simulink model "MBE_Simulation_04_Template_14_11_final"  (R2017b)
settings: Solver=FixedStepAuto  StartTime=0.0  StopTime=inf  FixedStep=0.05  RelTol=1e-3
libraries: simulink x67, canmsglib x4, instrumentlib x2, realtime_pacer_lib x1, hdlsllib x1
(part 2 of 4)

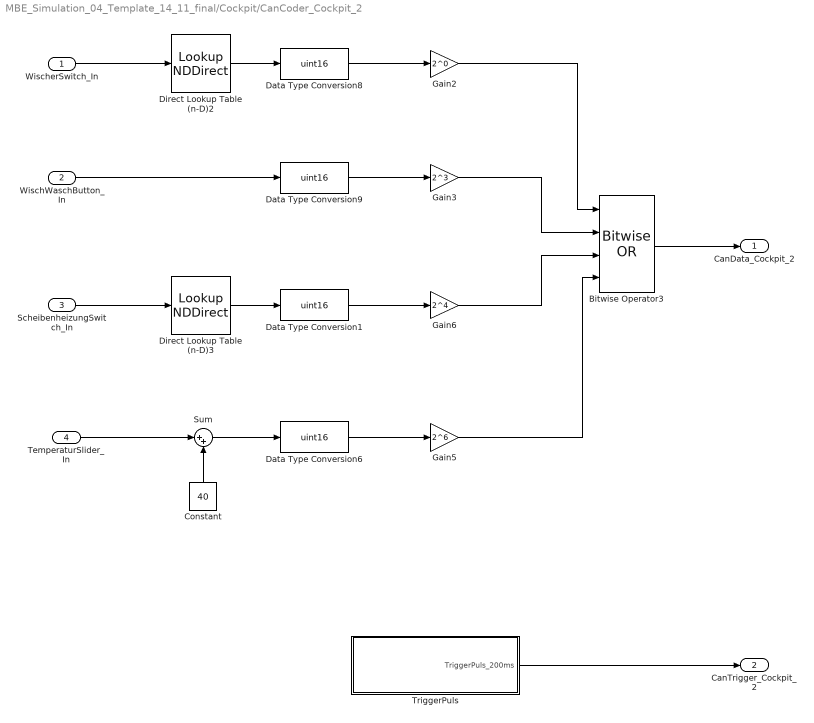
== system MBE_Simulation_04_Template_14_11_final/Cockpit/CanCoder_Cockpit_2 ==
  WischerSwitch_In : Inport
  WischWaschButton_In : Inport  Port=2
  ScheibenheizungSwitch_In : Inport  Port=3
  TemperaturSlider_In : Inport  Port=4
  Bitwise Operator3 : simulink/Logic and Bit Operations/Bitwise Operator  logicop=OR  UseBitMask=off  NumInputPorts=4  BitMask=bin2dec('11011001')  BitMaskRealWorld=Stored Integer
  Constant : Constant  Value=40  OutDataTypeStr=int16
  Data Type Conversion{1,6,8..9} (4 alike) : DataTypeConversion  OutDataTypeStr=uint16
  Direct Lookup Table (n-D)2 : LookupNDDirect  NumberOfTableDimensions=1  Table=[1; 0; 2; 3; 4; 5]
  Direct Lookup Table (n-D)3 : LookupNDDirect  NumberOfTableDimensions=1  Table=[1; 0; 2]
  Gain2 : Gain  Gain=2^0  OutDataTypeStr=uint16
  Gain3 : Gain  Gain=2^3  OutDataTypeStr=uint16
  Gain5 : Gain  Gain=2^6  OutDataTypeStr=uint16
  Gain6 : Gain  Gain=2^4  OutDataTypeStr=uint16
  Sum : Sum  Inputs=|++
  TriggerPuls : Subsystem
  CanData_Cockpit_2 : Outport
  CanTrigger_Cockpit_2 : Outport  Port=2
  wires:
  Data Type Conversion8/1 -> Gain2/1
  Sum/1 -> Data Type Conversion6/1
  Bitwise Operator3/1 -> CanData_Cockpit_2/1
  Data Type Conversion9/1 -> Gain3/1
  Constant/1 -> Sum/2
  Data Type Conversion6/1 -> Gain5/1
  Data Type Conversion1/1 -> Gain6/1
  Direct Lookup Table (n-D)2/1 -> Data Type Conversion8/1
  Direct Lookup Table (n-D)3/1 -> Data Type Conversion1/1
  Gain2/1 -> Bitwise Operator3/1
  Gain3/1 -> Bitwise Operator3/2
  Gain6/1 -> Bitwise Operator3/3
  Gain5/1 -> Bitwise Operator3/4
  ScheibenheizungSwitch_In/1 -> Direct Lookup Table (n-D)3/1
  TemperaturSlider_In/1 -> Sum/1
  WischWaschButton_In/1 -> Data Type Conversion9/1
  WischerSwitch_In/1 -> Direct Lookup Table (n-D)2/1
  TriggerPuls/1(TriggerPuls_200ms) -> CanTrigger_Cockpit_2/1

== system MBE_Simulation_04_Template_14_11_final/Cockpit/CanCoder_Cockpit_3 ==
  AlarmResetButton_In : Inport
  Detect Change4 : simulink/Logic and Bit Operations/Detect Change  vinit=0  OutDataTypeStr=boolean
  Gain : Gain  Gain=2^0  OutDataTypeStr=uint8
  CanData_Cockpit_3 : Outport
  CanTrigger_Cockpit_3 : Outport  Port=2
  wires:
  AlarmResetButton_In/1 -> Detect Change4/1, Gain/1
  Gain/1 -> CanData_Cockpit_3/1
  Detect Change4/1 -> CanTrigger_Cockpit_3/1

== system MBE_Simulation_04_Template_14_11_final/Cockpit/CanCoder_Cockpit_4 ==
  IgnitionSwitch_In : Inport
  Detect Change4 : simulink/Logic and Bit Operations/Detect Change  vinit=0  OutDataTypeStr=boolean
  Gain : Gain  Gain=2^0  OutDataTypeStr=uint8
  CanData_Cockpit_4 : Outport
  CanTrigger_Cockpit_4 : Outport  Port=2
  wires:
  Detect Change4/1 -> CanTrigger_Cockpit_4/1
  Gain/1 -> CanData_Cockpit_4/1
  IgnitionSwitch_In/1 -> Gain/1, Detect Change4/1

== system MBE_Simulation_04_Template_14_11_final/Cockpit/CanTransmit_Bremse_1 ==
  CanData_Bremse_1_In : Inport
  CanTrigger_Bremse_1_In : Inport  Port=2
  Bus Creator6 : BusCreator  Inputs=2
  CanTrigger_Bremse_1_Out : Outport
  wires:
  CanData_Bremse_1_In/1 -> Bus Creator6/1
  Bus Creator6/1 -> CanTrigger_Bremse_1_Out/1  "CanMsg_Bremse_1"
  CanTrigger_Bremse_1_In/1 -> Bus Creator6/2

== system MBE_Simulation_04_Template_14_11_final/Cockpit/CanTransmit_Bremse_2 ==
  CanData_Bremse_2_In : Inport
  CanTrigger_Bremse_2_In : Inport  Port=2
  Bus Creator3 : BusCreator  Inputs=2
  CanMsg_Bremse_2_Out : Outport
  wires:
  CanData_Bremse_2_In/1 -> Bus Creator3/1
  CanTrigger_Bremse_2_In/1 -> Bus Creator3/2
  Bus Creator3/1 -> CanMsg_Bremse_2_Out/1  "CanMsg_Bremse_2"

== system MBE_Simulation_04_Template_14_11_final/Cockpit/CanTransmit_Cockpit_1 ==
  CanData_Cockpit_1_In : Inport
  CanTrigger_Cockpit_1_In : Inport  Port=2
  Bus Creator : BusCreator  Inputs=2
  CanMsg_Cockpit_1_Out : Outport
  wires:
  CanData_Cockpit_1_In/1 -> Bus Creator/1
  CanTrigger_Cockpit_1_In/1 -> Bus Creator/2
  Bus Creator/1 -> CanMsg_Cockpit_1_Out/1  "CanMsg_Cockpit_1"

== system MBE_Simulation_04_Template_14_11_final/Cockpit/CanTransmit_Cockpit_2 ==
  CanData_Cockpit_2_In : Inport
  CanTrigger_Cockpit_2_In : Inport  Port=2
  Bus Creator1 : BusCreator  Inputs=2
  CanMsg_Cockpit_2_Out : Outport
  wires:
  CanData_Cockpit_2_In/1 -> Bus Creator1/1
  CanTrigger_Cockpit_2_In/1 -> Bus Creator1/2
  Bus Creator1/1 -> CanMsg_Cockpit_2_Out/1  "CanMsg_Cockpit_2"

== system MBE_Simulation_04_Template_14_11_final/Cockpit/CanTransmit_Cockpit_3 ==
  CanData_Cockpit_3_In : Inport
  CanTrigger_Cockpit_3_In : Inport  Port=2
  Bus Creator2 : BusCreator  Inputs=2
  CanMsg_Cockpit_3_Out : Outport
  wires:
  CanData_Cockpit_3_In/1 -> Bus Creator2/1
  CanTrigger_Cockpit_3_In/1 -> Bus Creator2/2
  Bus Creator2/1 -> CanMsg_Cockpit_3_Out/1  "CanMsg_Cockpit_3"

== system MBE_Simulation_04_Template_14_11_final/Cockpit/CanTransmit_Cockpit_4 ==
  CanData_Cockpit_4_In : Inport
  CanTrigger_Cockpit_4_In : Inport  Port=2
  Bus Creator5 : BusCreator  Inputs=2
  CanMsg_Cockpit_4_Out : Outport
  wires:
  CanData_Cockpit_4_In/1 -> Bus Creator5/1
  CanTrigger_Cockpit_4_In/1 -> Bus Creator5/2
  Bus Creator5/1 -> CanMsg_Cockpit_4_Out/1  "CanMsg_Cockpit_4"

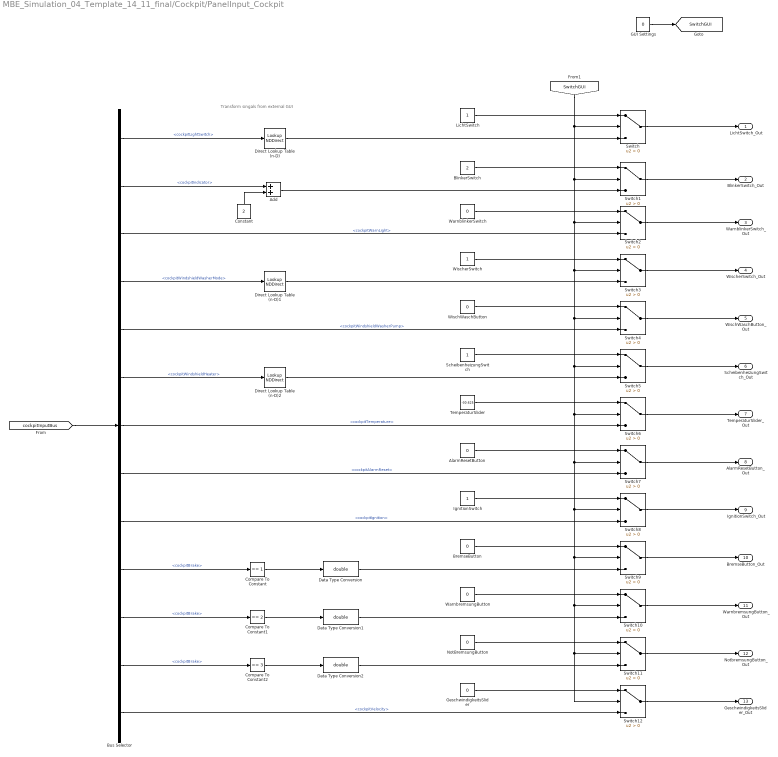
== system MBE_Simulation_04_Template_14_11_final/Cockpit/PanelInput_Cockpit ==
  note: Transform singals from external GUI
  Add : Sum
  AlarmResetButton : Constant  Value=0  OutDataTypeStr=uint8
  BlinkerSwitch : Constant  Value=2  OutDataTypeStr=uint8
  BremseButton : Constant  Value=0  OutDataTypeStr=uint8
  Bus Selector : BusSelector  OutputSignals=cockpitLightSwitch,cockpitIndicator,cockpitWarnLight,cockpitWindshieldWasherMode,cockpitWindshieldWasherPump,cockpitWindshieldHeater,cockpitTemperature,cockpitAlarmReset,cockpitIgnition,cockpitBrake,cockpitBrake,cockpitBrake,cockpitVelocity
  Compare To Constant : simulink/Logic and Bit Operations/Compare To Constant  relop===  const=1  OutDataTypeStr=boolean
  Compare To Constant1 : simulink/Logic and Bit Operations/Compare To Constant  relop===  const=2  OutDataTypeStr=boolean
  Compare To Constant2 : simulink/Logic and Bit Operations/Compare To Constant  relop===  const=3  OutDataTypeStr=boolean
  Constant : Constant  Value=2
  Data Type Conversion : DataTypeConversion  OutDataTypeStr=double
  Data Type Conversion1 : DataTypeConversion  OutDataTypeStr=double
  Data Type Conversion2 : DataTypeConversion  OutDataTypeStr=double
  Direct Lookup Table (n-D) : LookupNDDirect  NumberOfTableDimensions=1  Table=[1 0 2 3 4]
  Direct Lookup Table (n-D)1 : LookupNDDirect  NumberOfTableDimensions=1  Table=[1 0 2 3 4 5]
  Direct Lookup Table (n-D)2 : LookupNDDirect  NumberOfTableDimensions=1  Table=[1 0 2]
  GUI Settings : Constant  Value=0
  GeschwindigkeitsSlider : Constant  Value=0  OutDataTypeStr=uint8
  IgnitionSwitch : Constant  OutDataTypeStr=uint8
  LichtSwitch : Constant  OutDataTypeStr=uint8
  NotBremsungButton : Constant  Value=0  OutDataTypeStr=uint8
  ScheibenheizungSwitch : Constant  OutDataTypeStr=uint8
  Switch{,1..12} (13 alike) : Switch  Criteria=u2 > Threshold
  TemperaturSlider : Constant  Value=-30.625  OutDataTypeStr=int16
  WarnblinkerSwitch : Constant  Value=0  OutDataTypeStr=uint8
  WarnbremsungButton : Constant  Value=0  OutDataTypeStr=uint8
  WischWaschButton : Constant  Value=0  OutDataTypeStr=uint8
  WischerSwitch : Constant  OutDataTypeStr=uint8
  LichtSwitch_Out : Outport
  BlinkerSwitch_Out : Outport  Port=2
  WarnblinkerSwitch_Out : Outport  Port=3
  WischerSwitch_Out : Outport  Port=4
  WischWaschButton_Out : Outport  Port=5
  ScheibenheizungSwitch_Out : Outport  Port=6
  TemperaturSlider_Out : Outport  Port=7
  AlarmResetButton_Out : Outport  Port=8
  IgnitionSwitch_Out : Outport  Port=9
  BremseButton_Out : Outport  Port=10
  WarnbremsungButton_Out : Outport  Port=11
  NotbremsungButton_Out : Outport  Port=12
  GeschwindigkeitsSlider_Out : Outport  Port=13
  tag scope: SwitchGUI=global
  wires:
  [cockpitInputBus] -> Bus Selector/1
  Bus Selector/2 -> Add/1  "<cockpitIndicator>"
  Constant/1 -> Add/2
  Bus Selector/1 -> Direct Lookup Table (n-D)/1  "<cockpitLightSwitch>"
  Bus Selector/4 -> Direct Lookup Table (n-D)1/1  "<cockpitWindshieldWasherMode>"
  Bus Selector/10 -> Compare To Constant/1  "<cockpitBrake>"
  Bus Selector/6 -> Direct Lookup Table (n-D)2/1  "<cockpitWindshieldHeater>"
  Compare To Constant/1 -> Data Type Conversion/1
  Compare To Constant1/1 -> Data Type Conversion1/1
  Compare To Constant2/1 -> Data Type Conversion2/1
  Bus Selector/11 -> Compare To Constant1/1  "<cockpitBrake>"
  Bus Selector/12 -> Compare To Constant2/1  "<cockpitBrake>"
  Direct Lookup Table (n-D)/1 -> Switch/3
  Add/1 -> Switch1/3
  Bus Selector/3 -> Switch2/3  "<cockpitWarnLight>"
  Direct Lookup Table (n-D)1/1 -> Switch3/3
  Bus Selector/5 -> Switch4/3  "<cockpitWindshieldWasherPump>"
  Direct Lookup Table (n-D)2/1 -> Switch5/3
  Bus Selector/7 -> Switch6/3  "<cockpitTemperature>"
  Bus Selector/8 -> Switch7/3  "<cockpitAlarmReset>"
  Bus Selector/9 -> Switch8/3  "<cockpitIgnition>"
  Data Type Conversion/1 -> Switch9/3
  Data Type Conversion1/1 -> Switch10/3
  Data Type Conversion2/1 -> Switch11/3
  Bus Selector/13 -> Switch12/3  "<cockpitVelocity>"
  LichtSwitch/1 -> Switch/1
  BlinkerSwitch/1 -> Switch1/1
  WarnblinkerSwitch/1 -> Switch2/1
  WischerSwitch/1 -> Switch3/1
  WischWaschButton/1 -> Switch4/1
  ScheibenheizungSwitch/1 -> Switch5/1
  TemperaturSlider/1 -> Switch6/1
  AlarmResetButton/1 -> Switch7/1
  IgnitionSwitch/1 -> Switch8/1
  BremseButton/1 -> Switch9/1
  WarnbremsungButton/1 -> Switch10/1
  NotBremsungButton/1 -> Switch11/1
  GeschwindigkeitsSlider/1 -> Switch12/1
  Switch/1 -> LichtSwitch_Out/1
  Switch1/1 -> BlinkerSwitch_Out/1
  Switch2/1 -> WarnblinkerSwitch_Out/1
  Switch3/1 -> WischerSwitch_Out/1
  Switch4/1 -> WischWaschButton_Out/1
  Switch5/1 -> ScheibenheizungSwitch_Out/1
  Switch6/1 -> TemperaturSlider_Out/1
  Switch7/1 -> AlarmResetButton_Out/1
  Switch8/1 -> IgnitionSwitch_Out/1
  Switch9/1 -> BremseButton_Out/1
  Switch10/1 -> WarnbremsungButton_Out/1
  Switch11/1 -> NotbremsungButton_Out/1
  Switch12/1 -> GeschwindigkeitsSlider_Out/1
  [SwitchGUI] -> Switch/2, Switch1/2, Switch2/2, Switch3/2, Switch4/2, Switch5/2, Switch6/2, Switch7/2, Switch8/2, Switch9/2, Switch10/2, Switch11/2, Switch12/2
  GUI Settings/1 -> [SwitchGUI]

== system MBE_Simulation_04_Template_14_11_final/Dashboard/Gauge ==

== system MBE_Simulation_04_Template_14_11_final/Dashboard/Lamp ==

== system MBE_Simulation_04_Template_14_11_final/Dashboard/Lamp1 ==

== system MBE_Simulation_04_Template_14_11_final/Dashboard/Lamp10 ==

== system MBE_Simulation_04_Template_14_11_final/Dashboard/Lamp11 ==

== system MBE_Simulation_04_Template_14_11_final/Dashboard/Lamp12 ==

== system MBE_Simulation_04_Template_14_11_final/Dashboard/Lamp13 ==

== system MBE_Simulation_04_Template_14_11_final/Dashboard/Lamp14 ==

== system MBE_Simulation_04_Template_14_11_final/Dashboard/Lamp15 ==

== system MBE_Simulation_04_Template_14_11_final/Dashboard/Lamp16 ==

== system MBE_Simulation_04_Template_14_11_final/Dashboard/Lamp17 ==

== system MBE_Simulation_04_Template_14_11_final/Dashboard/Lamp18 ==

== system MBE_Simulation_04_Template_14_11_final/Dashboard/Lamp2 ==

== system MBE_Simulation_04_Template_14_11_final/Dashboard/Lamp20 ==

== system MBE_Simulation_04_Template_14_11_final/Dashboard/Lamp3 ==

== system MBE_Simulation_04_Template_14_11_final/Dashboard/Lamp4 ==

== system MBE_Simulation_04_Template_14_11_final/Dashboard/Lamp5 ==

== system MBE_Simulation_04_Template_14_11_final/Dashboard/Lamp6 ==

== system MBE_Simulation_04_Template_14_11_final/Dashboard/Lamp7 ==

== system MBE_Simulation_04_Template_14_11_final/Dashboard/Lamp8 ==

== system MBE_Simulation_04_Template_14_11_final/Dashboard/Lamp9 ==

== system MBE_Simulation_04_Template_14_11_final/Dashboard/Push Button ==

== system MBE_Simulation_04_Template_14_11_final/Dashboard/Push Button1 ==

== system MBE_Simulation_04_Template_14_11_final/Dashboard/Push Button2 ==

== system MBE_Simulation_04_Template_14_11_final/Dashboard/Push Button4 ==

== system MBE_Simulation_04_Template_14_11_final/Dashboard/Push Button5 ==

== system MBE_Simulation_04_Template_14_11_final/Dashboard/Quarter Gauge ==

== system MBE_Simulation_04_Template_14_11_final/Dashboard/Rocker Switch ==

== system MBE_Simulation_04_Template_14_11_final/Dashboard/Rocker Switch6 ==

== system MBE_Simulation_04_Template_14_11_final/Dashboard/Rotary Switch ==

== system MBE_Simulation_04_Template_14_11_final/Dashboard/Rotary Switch1 ==

== system MBE_Simulation_04_Template_14_11_final/Dashboard/Rotary Switch2 ==

== system MBE_Simulation_04_Template_14_11_final/Dashboard/Rotary Switch3 ==

== system MBE_Simulation_04_Template_14_11_final/Dashboard/Slider ==

== system MBE_Simulation_04_Template_14_11_final/Dashboard/Slider1 ==

== system MBE_Simulation_04_Template_14_11_final/Dashboard/Slider2 ==

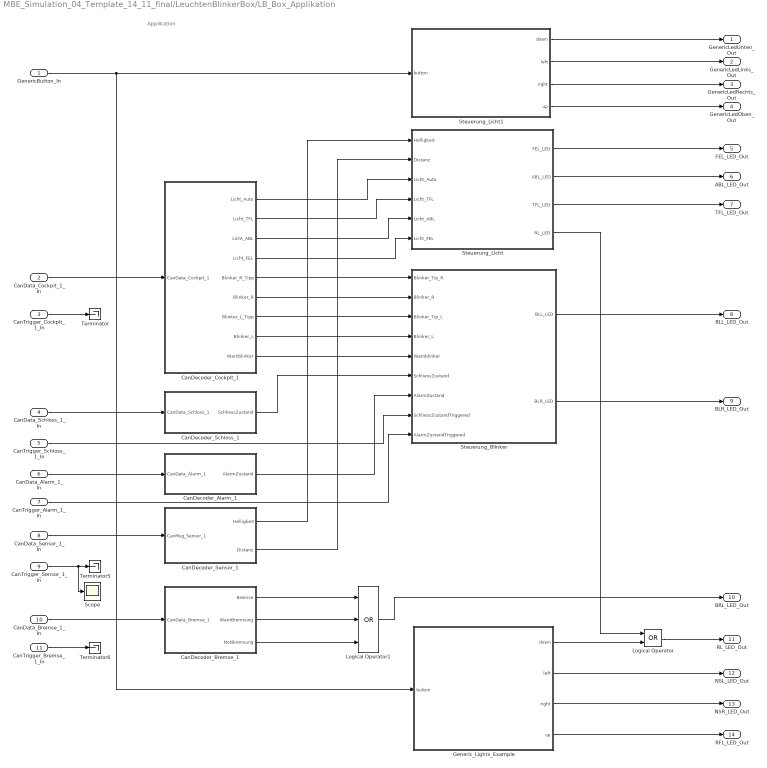
== system MBE_Simulation_04_Template_14_11_final/LeuchtenBlinkerBox/LB_Box_Applikation ==
  note: Applikation
  GenericButton_In : Inport
  CanData_Cockpit_1_In : Inport  Port=2
  CanTrigger_Cockpit_1_In : Inport  Port=3
  CanData_Schloss_1_In : Inport  Port=4
  CanTrigger_Schloss_1_In : Inport  Port=5
  CanData_Alarm_1_In : Inport  Port=6
  CanTrigger_Alarm_1_In : Inport  Port=7
  CanData_Sensor_1_In : Inport  Port=8
  CanTrigger_Sensor_1_In : Inport  Port=9
  CanData_Bremse_1_In : Inport  Port=10
  CanTrigger_Bremse_1_In : Inport  Port=11
  CanDecoder_Alarm_1 : Subsystem
  CanDecoder_Bremse_1 : Subsystem
  CanDecoder_Cockpit_1 : Subsystem
  CanDecoder_Schloss_1 : Subsystem
  CanDecoder_Sensor_1 : Subsystem
  Generic_Lights_Example : Stateflow chart  TreatAsAtomicUnit=on
  Logical Operator : Logic  Operator=OR  AllPortsSameDT=off  OutDataTypeStr=boolean
  Logical Operator1 : Logic  Operator=OR  Inputs=3  AllPortsSameDT=off  OutDataTypeStr=boolean
  Scope : Scope
  Steuerung_Blinker : Stateflow chart  TreatAsAtomicUnit=on
  Steuerung_Licht : Stateflow chart  TreatAsAtomicUnit=on
  Steuerung_Licht1 : Stateflow chart  TreatAsAtomicUnit=on
  Terminator : Terminator
  Terminator5 : Terminator
  Terminator6 : Terminator
  GenericLedUnten_Out : Outport
  GenericLedLinks_Out : Outport  Port=2
  GenericLedRechts_Out : Outport  Port=3
  GenericLedOben_Out : Outport  Port=4
  FEL_LED_Out : Outport  Port=5
  ABL_LED_Out : Outport  Port=6
  TFL_LED_Out : Outport  Port=7
  BLL_LED_Out : Outport  Port=8
  BLR_LED_Out : Outport  Port=9
  BRL_LED_Out : Outport  Port=10
  RL_LED_Out : Outport  Port=11
  NSL_LED_Out : Outport  Port=12
  NSR_LED_Out : Outport  Port=13
  RFL_LED_Out : Outport  Port=14
  wires:
  Steuerung_Blinker/2(BLR_LED) -> BLR_LED_Out/1
  Steuerung_Licht/2(ABL_LED) -> ABL_LED_Out/1
  Steuerung_Blinker/1(BLL_LED) -> BLL_LED_Out/1
  CanDecoder_Bremse_1/2(WarnBremsung) -> Logical Operator1/2
  CanDecoder_Cockpit_1/9(Warnblinker) -> Steuerung_Blinker/5(Warnblinker)
  CanDecoder_Cockpit_1/3(Licht_ABL) -> Steuerung_Licht/5(Licht_ABL)
  CanDecoder_Sensor_1/1(Helligkeit) -> Steuerung_Licht/1(Helligkeit)
  CanDecoder_Cockpit_1/4(Licht_FEL) -> Steuerung_Licht/6(Licht_FEL)
  CanDecoder_Cockpit_1/5(Blinker_R_Tipp) -> Steuerung_Blinker/1(Blinker_Tip_R)
  CanDecoder_Cockpit_1/8(Blinker_L) -> Steuerung_Blinker/4(Blinker_L)
  CanDecoder_Schloss_1/1(SchliessZustand) -> Steuerung_Blinker/6(SchliessZustand)
  CanDecoder_Alarm_1/1(AlarmZustand) -> Steuerung_Blinker/7(AlarmZustand)
  CanDecoder_Cockpit_1/1(Licht_Auto) -> Steuerung_Licht/3(Licht_Auto)
  CanDecoder_Cockpit_1/6(Blinker_R) -> Steuerung_Blinker/2(Blinker_R)
  CanDecoder_Cockpit_1/2(Licht_TFL) -> Steuerung_Licht/4(Licht_TFL)
  CanDecoder_Sensor_1/2(Distanz) -> Steuerung_Licht/2(Distanz)
  CanDecoder_Cockpit_1/7(Blinker_L_Tipp) -> Steuerung_Blinker/3(Blinker_Tip_L)
  CanData_Sensor_1_In/1 -> CanDecoder_Sensor_1/1(CanMsg_Sensor_1)
  CanData_Cockpit_1_In/1 -> CanDecoder_Cockpit_1/1(CanData_Cockpit_1)
  CanData_Schloss_1_In/1 -> CanDecoder_Schloss_1/1(CanData_Schloss_1)
  CanData_Alarm_1_In/1 -> CanDecoder_Alarm_1/1(CanData_Alarm_1)
  CanData_Bremse_1_In/1 -> CanDecoder_Bremse_1/1(CanData_Bremse_1)
  CanTrigger_Cockpit_1_In/1 -> Terminator/1
  CanTrigger_Schloss_1_In/1 -> Steuerung_Blinker/8(SchliessZustandTriggered)
  CanTrigger_Alarm_1_In/1 -> Steuerung_Blinker/9(AlarmZustandTriggered)
  CanTrigger_Sensor_1_In/1 -> Scope/1, Terminator5/1
  CanTrigger_Bremse_1_In/1 -> Terminator6/1
  Steuerung_Licht/1(FEL_LED) -> FEL_LED_Out/1
  Steuerung_Licht/3(TFL_LED) -> TFL_LED_Out/1
  Steuerung_Licht1/1(down) -> GenericLedUnten_Out/1
  Steuerung_Licht1/2(left) -> GenericLedLinks_Out/1
  Steuerung_Licht1/3(right) -> GenericLedRechts_Out/1
  Steuerung_Licht1/4(up) -> GenericLedOben_Out/1
  GenericButton_In/1 -> Generic_Lights_Example/1(button), Steuerung_Licht1/1(button)
  Generic_Lights_Example/1(down) -> Logical Operator/2
  Generic_Lights_Example/2(left) -> NSL_LED_Out/1
  Generic_Lights_Example/3(right) -> NSR_LED_Out/1
  Generic_Lights_Example/4(up) -> RFL_LED_Out/1
  CanDecoder_Bremse_1/3(NotBremsung) -> Logical Operator1/3
  Steuerung_Licht/4(RL_LED) -> Logical Operator/1
  Logical Operator/1 -> RL_LED_Out/1
  CanDecoder_Bremse_1/1(Bremse) -> Logical Operator1/1
  Logical Operator1/1 -> BRL_LED_Out/1

== system MBE_Simulation_04_Template_14_11_final/LeuchtenBlinkerBox/LB_Box_Simulation_Input ==
  CanBus_LB_In : Inport
  CanBus_Input : Subsystem
  CanReceive_Alarm_1 : Subsystem
  CanReceive_Bremse_1 : Subsystem
  CanReceive_Cockpit_1 : Subsystem
  CanReceive_Schloss_1 : Subsystem
  CanReceive_Sensor_1 : Subsystem
  GuiInput_LichtBox : Subsystem
  GenericButton_Out : Outport
  CanData_Cockpit_1_Out : Outport  Port=2
  CanTrigger_Cockpit_1_Out : Outport  Port=3
  CanData_Schloss_1_Out : Outport  Port=4
  CanTrigger_Schloss_1_Out : Outport  Port=5
  CanData_Alarm_1_Out : Outport  Port=6
  CanTrigger_Alarm_1_Out : Outport  Port=7
  CanData_Sensor_1_Out : Outport  Port=8
  CanTrigger_Sensor_1_Out : Outport  Port=9
  CanData_Bremse_1_Out : Outport  Port=10
  CanTrigger_Bremse_1_Out : Outport  Port=11
  wires:
  CanBus_LB_In/1 -> CanBus_Input/1(CanBus_LB_In)
  CanBus_Input/1(CanMsg_Cockpit_1_Out) -> CanReceive_Cockpit_1/1(CanData_Cockpit_1_In)
  CanBus_Input/2(CanMsg_Schloss_1_Out) -> CanReceive_Schloss_1/1(CanMsg_Schloss_1_In)
  CanBus_Input/3(CanMsg_Alarm_1_Out) -> CanReceive_Alarm_1/1(CanMsg_Alarm_1_In)
  CanBus_Input/4(CanMsg_Sensor_1_Out) -> CanReceive_Sensor_1/1(CanMsg_Sensor_1_In)
  CanBus_Input/5(CanMsg_Bremse_1_Out) -> CanReceive_Bremse_1/1(CanMsg_Bremse_1_In)
  CanReceive_Sensor_1/1(CanData_Sensor_1_Out) -> CanData_Sensor_1_Out/1
  CanReceive_Cockpit_1/2(CanTrigger_Cockpit_1_Out) -> CanTrigger_Cockpit_1_Out/1
  CanReceive_Alarm_1/1(CanData_Alarm_1_Out) -> CanData_Alarm_1_Out/1
  CanReceive_Schloss_1/2(CanTrigger_Schloss_1_Out) -> CanTrigger_Schloss_1_Out/1
  CanReceive_Bremse_1/1(CanData_Bremse_1_Out) -> CanData_Bremse_1_Out/1
  CanReceive_Bremse_1/2(CanTrigger_Bremse_1_Out) -> CanTrigger_Bremse_1_Out/1
  CanReceive_Schloss_1/1(CanData_Schloss_1_Out) -> CanData_Schloss_1_Out/1
  CanReceive_Cockpit_1/1(CanData_Cockpit_1_Out) -> CanData_Cockpit_1_Out/1
  CanReceive_Sensor_1/2(CanTrigger_Sensor_1_Out) -> CanTrigger_Sensor_1_Out/1
  CanReceive_Alarm_1/2(CanTrigger_Alarm_1_Out) -> CanTrigger_Alarm_1_Out/1
  GuiInput_LichtBox/1(GenericButton_Out) -> GenericButton_Out/1

== system MBE_Simulation_04_Template_14_11_final/LeuchtenBlinkerBox/LB_Box_Simulation_Output ==
  GenericLedUnten_LED_In : Inport
  GenericLedLinks_LED_In : Inport  Port=2
  GenericLedRechts_LED_In : Inport  Port=3
  GenericLedOben_LED_In : Inport  Port=4
  FEL_LED : Inport  Port=5
  ABL_LED : Inport  Port=6
  TFL_LED : Inport  Port=7
  BLL_LED : Inport  Port=8
  BLR_LED : Inport  Port=9
  BRL_LED : Inport  Port=10
  RL_LED : Inport  Port=11
  NSL_LED : Inport  Port=12
  NSR_LED : Inport  Port=13
  RFL_LED : Inport  Port=14
  Bus Creator : BusCreator  Inputs=14
  LeuchtenBlinkerLEDs : Subsystem
  tag scope: lightOutputBus=global
  wires:
  FEL_LED/1 -> Bus Creator/5, LeuchtenBlinkerLEDs/1(FEL_LED)
  ABL_LED/1 -> Bus Creator/6, LeuchtenBlinkerLEDs/2(ABL_LED)
  TFL_LED/1 -> Bus Creator/7, LeuchtenBlinkerLEDs/3(TFL_LED)
  BLL_LED/1 -> Bus Creator/8, LeuchtenBlinkerLEDs/4(BLL_LED)
  BLR_LED/1 -> Bus Creator/9, LeuchtenBlinkerLEDs/5(BLR_LED)
  BRL_LED/1 -> Bus Creator/10, LeuchtenBlinkerLEDs/6(BRL_LED)  "BRL_LED"
  Bus Creator/1 -> [lightOutputBus]
  GenericLedOben_LED_In/1 -> Bus Creator/4  "GenericLedOben"
  GenericLedRechts_LED_In/1 -> Bus Creator/3  "GenericLedRechts"
  GenericLedLinks_LED_In/1 -> Bus Creator/2  "GenericLedLinks"
  GenericLedUnten_LED_In/1 -> Bus Creator/1  "GenericLedUnten"
  RL_LED/1 -> Bus Creator/11  "RL_LED"
  NSL_LED/1 -> Bus Creator/12  "NSL_LED"
  NSR_LED/1 -> Bus Creator/13  "NSR_LED"
  RFL_LED/1 -> Bus Creator/14  "RFL_LED"

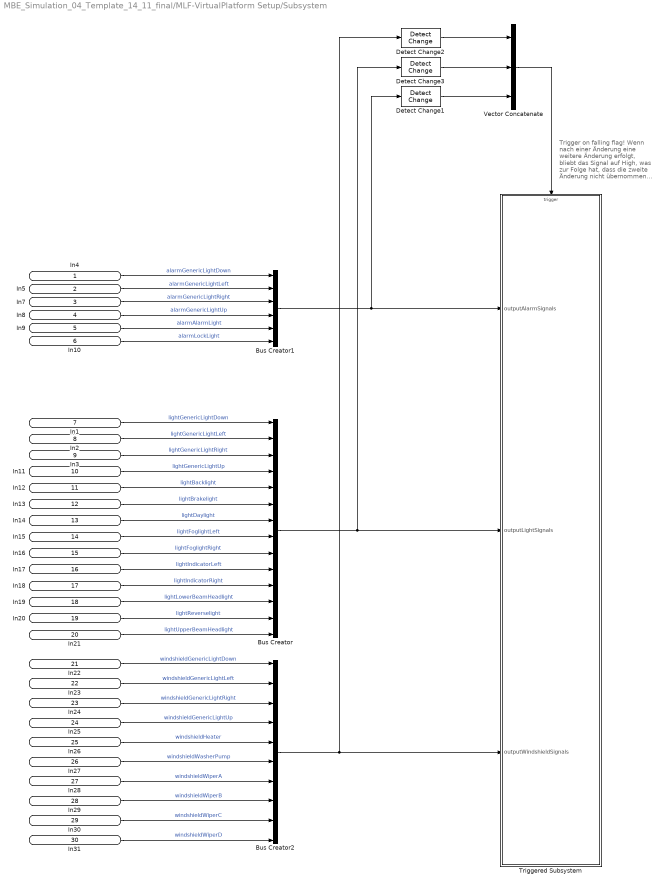
== system MBE_Simulation_04_Template_14_11_final/MLF-VirtualPlatform Setup/Subsystem ==
  note: Trigger on falling flag!
      | Wenn nach einer Änderung eine weitere Änderung erfolgt,
      | bliebt das Signal auf High, was zur Folge hat, dass die zweite
      | Änderung nicht übernommen wird. Durch das Triggern auf eine
      | fallende Flanke erfolgt das übertragen erst dann, wenn sich für
      | mindestens ein Zeitschritt ein konstanter Zustand eingestellt hat.
  In4 : Inport
  In5 : Inport  Port=2
  In7 : Inport  Port=3
  In8 : Inport  Port=4
  In9 : Inport  Port=5
  In10 : Inport  Port=6
  In1 : Inport  Port=7
  In2 : Inport  Port=8
  In3 : Inport  Port=9
  In11 : Inport  Port=10
  In12 : Inport  Port=11
  In13 : Inport  Port=12
  In14 : Inport  Port=13
  In15 : Inport  Port=14
  In16 : Inport  Port=15
  In17 : Inport  Port=16
  In18 : Inport  Port=17
  In19 : Inport  Port=18
  In20 : Inport  Port=19
  In21 : Inport  Port=20
  In22 : Inport  Port=21
  In23 : Inport  Port=22
  In24 : Inport  Port=23
  In25 : Inport  Port=24
  In26 : Inport  Port=25
  In27 : Inport  Port=26
  In28 : Inport  Port=27
  In29 : Inport  Port=28
  In30 : Inport  Port=29
  In31 : Inport  Port=30
  Bus Creator : BusCreator  Inputs=14
  Bus Creator1 : BusCreator  Inputs=6
  Bus Creator2 : BusCreator  Inputs=10
  Detect Change1 : simulink/Logic and Bit Operations/Detect Change  vinit=0  OutDataTypeStr=boolean
  Detect Change2 : simulink/Logic and Bit Operations/Detect Change  vinit=0  OutDataTypeStr=boolean
  Detect Change3 : simulink/Logic and Bit Operations/Detect Change  vinit=0  OutDataTypeStr=boolean
  Triggered Subsystem : Subsystem  TreatAsAtomicUnit=on
  Vector Concatenate : Concatenate  NumInputs=3
  wires:
  Bus Creator/1 -> Detect Change3/1, Triggered Subsystem/2("outputLightSignals ")
  In1/1 -> Bus Creator/1  "lightGenericLightDown"
  In2/1 -> Bus Creator/2  "lightGenericLightLeft"
  In3/1 -> Bus Creator/3  "lightGenericLightRight"
  Detect Change3/1 -> Vector Concatenate/2
  In4/1 -> Bus Creator1/1  "alarmGenericLightDown"
  In5/1 -> Bus Creator1/2  "alarmGenericLightLeft"
  Bus Creator1/1 -> Detect Change1/1, Triggered Subsystem/1(outputAlarmSignals)
  Detect Change1/1 -> Vector Concatenate/3
  Vector Concatenate/1 -> Triggered Subsystem/Trigger
  In7/1 -> Bus Creator1/3  "alarmGenericLightRight"
  In8/1 -> Bus Creator1/4  "alarmGenericLightUp"
  In9/1 -> Bus Creator1/5  "alarmAlarmLight"
  In10/1 -> Bus Creator1/6  "alarmLockLight"
  Bus Creator2/1 -> Detect Change2/1, Triggered Subsystem/3(outputWindshieldSignals)
  Detect Change2/1 -> Vector Concatenate/1
  In11/1 -> Bus Creator/4  "lightGenericLightUp"
  In12/1 -> Bus Creator/5  "lightBacklight"
  In13/1 -> Bus Creator/6  "lightBrakelight"
  In14/1 -> Bus Creator/7  "lightDaylight"
  In15/1 -> Bus Creator/8  "lightFoglightLeft"
  In16/1 -> Bus Creator/9  "lightFoglightRight"
  In17/1 -> Bus Creator/10  "lightIndicatorLeft"
  In18/1 -> Bus Creator/11  "lightIndicatorRight"
  In19/1 -> Bus Creator/12  "lightLowerBeamHeadlight"
  In21/1 -> Bus Creator/14  "lightUpperBeamHeadlight"
  In20/1 -> Bus Creator/13  "lightReverselight"
  In22/1 -> Bus Creator2/1  "windshieldGenericLightDown"
  In23/1 -> Bus Creator2/2  "windshieldGenericLightLeft"
  In24/1 -> Bus Creator2/3  "windshieldGenericLightRight"
  In25/1 -> Bus Creator2/4  "windshieldGenericLightUp"
  In26/1 -> Bus Creator2/5  "windshieldHeater"
  In27/1 -> Bus Creator2/6  "windshieldWasherPump"
  In28/1 -> Bus Creator2/7  "windshieldWiperA"
  In29/1 -> Bus Creator2/8  "windshieldWiperB"
  In30/1 -> Bus Creator2/9  "windshieldWiperC"
  In31/1 -> Bus Creator2/10  "windshieldWiperD"

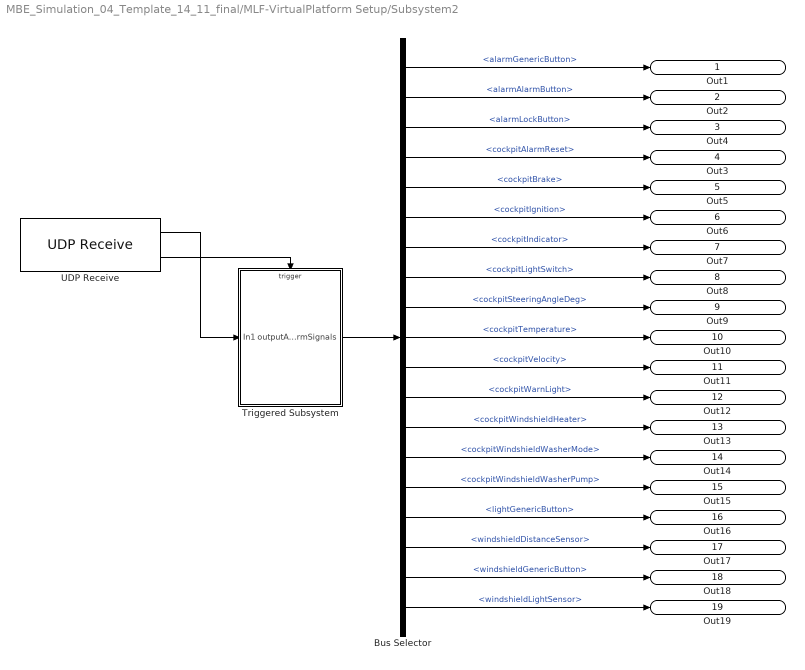
== system MBE_Simulation_04_Template_14_11_final/MLF-VirtualPlatform Setup/Subsystem2 ==
  Bus Selector : BusSelector  OutputSignals=alarmGenericButton,alarmAlarmButton,alarmLockButton,cockpitAlarmReset,cockpitBrake,cockpitIgnition,cockpitIndicator,cockpitLightSwitch,cockpitSteeringAngleDeg,cockpitTemperature,cockpitVelocity,cockpitWarnLight,cockpitWindshieldHeater,cockpitWindshieldWasherMode,cockpitWindshieldWasherPump,lightGenericButton,windshieldDistanceSensor,windshieldGenericButton,windshieldLightSensor
  Triggered Subsystem : Subsystem  TreatAsAtomicUnit=on
  UDP Receive : instrumentlib/UDP Receive  Host=127.0.0.1  Port=50001  LocalPort=50001  DataSize=4096  EnableBlockingMode=off  Timeout=10  SampleTime=0.05  DataType=uint8  ByteOrder=BigEndian
      settings: SourceProductName=Instrument Control Toolbox
  Out1 : Outport
  Out2 : Outport  Port=2
  Out4 : Outport  Port=3
  Out3 : Outport  Port=4
  Out5 : Outport  Port=5
  Out6 : Outport  Port=6
  Out7 : Outport  Port=7
  Out8 : Outport  Port=8
  Out9 : Outport  Port=9
  Out10 : Outport  Port=10
  Out11 : Outport  Port=11
  Out12 : Outport  Port=12
  Out13 : Outport  Port=13
  Out14 : Outport  Port=14
  Out15 : Outport  Port=15
  Out16 : Outport  Port=16
  Out17 : Outport  Port=17
  Out18 : Outport  Port=18
  Out19 : Outport  Port=19
  wires:
  UDP Receive/2 -> Triggered Subsystem/Trigger
  UDP Receive/1 -> Triggered Subsystem/1(In1)
  Triggered Subsystem/1(outputAlarmSignals) -> Bus Selector/1
  Bus Selector/1 -> Out1/1  "<alarmGenericButton>"
  Bus Selector/2 -> Out2/1  "<alarmAlarmButton>"
  Bus Selector/3 -> Out4/1  "<alarmLockButton>"
  Bus Selector/4 -> Out3/1  "<cockpitAlarmReset>"
  Bus Selector/5 -> Out5/1  "<cockpitBrake>"
  Bus Selector/6 -> Out6/1  "<cockpitIgnition>"
  Bus Selector/7 -> Out7/1  "<cockpitIndicator>"
  Bus Selector/19 -> Out19/1  "<windshieldLightSensor>"
  Bus Selector/18 -> Out18/1  "<windshieldGenericButton>"
  Bus Selector/17 -> Out17/1  "<windshieldDistanceSensor>"
  Bus Selector/16 -> Out16/1  "<lightGenericButton>"
  Bus Selector/15 -> Out15/1  "<cockpitWindshieldWasherPump>"
  Bus Selector/14 -> Out14/1  "<cockpitWindshieldWasherMode>"
  Bus Selector/13 -> Out13/1  "<cockpitWindshieldHeater>"
  Bus Selector/12 -> Out12/1  "<cockpitWarnLight>"
  Bus Selector/11 -> Out11/1  "<cockpitVelocity>"
  Bus Selector/10 -> Out10/1  "<cockpitTemperature>"
  Bus Selector/9 -> Out9/1  "<cockpitSteeringAngleDeg>"
  Bus Selector/8 -> Out8/1  "<cockpitLightSwitch>"

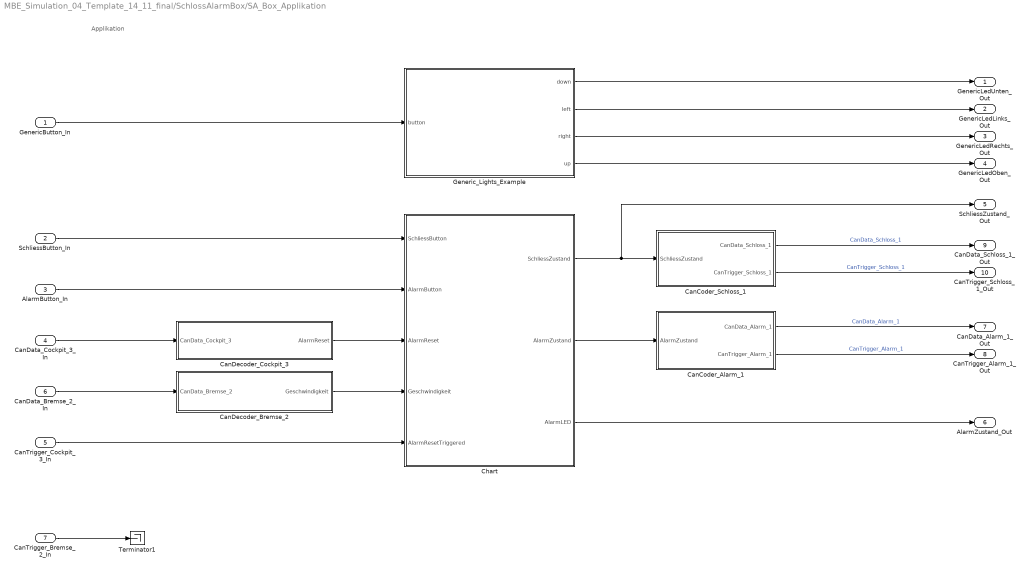
== system MBE_Simulation_04_Template_14_11_final/SchlossAlarmBox/SA_Box_Applikation ==
  note: Applikation
  GenericButton_In : Inport
  SchliessButton_In : Inport  Port=2
  AlarmButton_In : Inport  Port=3
  CanData_Cockpit_3_In : Inport  Port=4
  CanTrigger_Cockpit_3_In : Inport  Port=5
  CanData_Bremse_2_In : Inport  Port=6
  CanTrigger_Bremse_2_In : Inport  Port=7
  CanCoder_Alarm_1 : Subsystem
  CanCoder_Schloss_1 : Subsystem
  CanDecoder_Bremse_2 : Subsystem
  CanDecoder_Cockpit_3 : Subsystem
  Chart : Stateflow chart  TreatAsAtomicUnit=on
  Generic_Lights_Example : Stateflow chart  TreatAsAtomicUnit=on
  Terminator1 : Terminator
  GenericLedUnten_Out : Outport
  GenericLedLinks_Out : Outport  Port=2
  GenericLedRechts_Out : Outport  Port=3
  GenericLedOben_Out : Outport  Port=4
  SchliessZustand_Out : Outport  Port=5
  AlarmZustand_Out : Outport  Port=6
  CanData_Alarm_1_Out : Outport  Port=7
  CanTrigger_Alarm_1_Out : Outport  Port=8
  CanData_Schloss_1_Out : Outport  Port=9
  CanTrigger_Schloss_1_Out : Outport  Port=10
  wires:
  CanCoder_Schloss_1/1(CanData_Schloss_1) -> CanData_Schloss_1_Out/1  "CanData_Schloss_1"
  CanCoder_Alarm_1/1(CanData_Alarm_1) -> CanData_Alarm_1_Out/1  "CanData_Alarm_1"
  CanCoder_Alarm_1/2(CanTrigger_Alarm_1) -> CanTrigger_Alarm_1_Out/1  "CanTrigger_Alarm_1"
  CanCoder_Schloss_1/2(CanTrigger_Schloss_1) -> CanTrigger_Schloss_1_Out/1  "CanTrigger_Schloss_1"
  CanDecoder_Cockpit_3/1(AlarmReset) -> Chart/3(AlarmReset)
  CanDecoder_Bremse_2/1(Geschwindigkeit) -> Chart/4(Geschwindigkeit)
  Chart/2(AlarmZustand) -> CanCoder_Alarm_1/1(AlarmZustand)
  CanData_Cockpit_3_In/1 -> CanDecoder_Cockpit_3/1(CanData_Cockpit_3)
  SchliessButton_In/1 -> Chart/1(SchliessButton)
  CanData_Bremse_2_In/1 -> CanDecoder_Bremse_2/1(CanData_Bremse_2)
  AlarmButton_In/1 -> Chart/2(AlarmButton)
  CanTrigger_Cockpit_3_In/1 -> Chart/5(AlarmResetTriggered)
  CanTrigger_Bremse_2_In/1 -> Terminator1/1
  GenericButton_In/1 -> Generic_Lights_Example/1(button)
  Generic_Lights_Example/1(down) -> GenericLedUnten_Out/1
  Generic_Lights_Example/2(left) -> GenericLedLinks_Out/1
  Generic_Lights_Example/3(right) -> GenericLedRechts_Out/1
  Generic_Lights_Example/4(up) -> GenericLedOben_Out/1
  Chart/3(AlarmLED) -> AlarmZustand_Out/1
  Chart/1(SchliessZustand) -> SchliessZustand_Out/1, CanCoder_Schloss_1/1(SchliessZustand)

== system MBE_Simulation_04_Template_14_11_final/SchlossAlarmBox/SA_Box_Simulation_Input ==
  CanBus_SA_In : Inport
  CanBus_Input : Subsystem
  CanReceive_Bremse_2 : Subsystem
  CanReceive_Cockpit_3 : Subsystem
  PanelInput_SchlossAlarmBox : Subsystem
  GenericButton_Out : Outport
  SchliessButton_Out : Outport  Port=2
  AlarmButton_Out : Outport  Port=3
  CanData_Cockpit_3_Out : Outport  Port=4
  CanTrigger_Cockpit_3_Out : Outport  Port=5
  CanData_Bremse_2_Out : Outport  Port=6
  CanTrigger_Bremse_2_Out : Outport  Port=7
  wires:
  CanBus_Input/1(CanMsg_Cockpit_3_Out) -> CanReceive_Cockpit_3/1(CanMsg_Cockpit_3_In)
  CanReceive_Bremse_2/2(CanTrigger_Bremse_2_Out) -> CanTrigger_Bremse_2_Out/1
  CanBus_SA_In/1 -> CanBus_Input/1(CanBus_SA_In)
  CanReceive_Cockpit_3/2(CanTrigger_Cockpit_3_Out) -> CanTrigger_Cockpit_3_Out/1
  CanReceive_Bremse_2/1(CanData_Bremse_2_Out) -> CanData_Bremse_2_Out/1
  CanReceive_Cockpit_3/1(CanData_Cockpit_3_Out) -> CanData_Cockpit_3_Out/1
  PanelInput_SchlossAlarmBox/3(AlarmButton_Out) -> AlarmButton_Out/1
  PanelInput_SchlossAlarmBox/2(SchliessButton_Out) -> SchliessButton_Out/1
  CanBus_Input/2(CanMsg_Bremse_2_Out) -> CanReceive_Bremse_2/1(CanMsg_Bremse_2_In)
  PanelInput_SchlossAlarmBox/1(GenericButton_Out) -> GenericButton_Out/1

== system MBE_Simulation_04_Template_14_11_final/SchlossAlarmBox/SA_Box_Simulation_Output ==
  GenericLedUnten_LED_In : Inport
  GenericLedLinks_LED_In : Inport  Port=2
  GenericLedRechts_LED_In : Inport  Port=3
  GenericLedOben_LED_In : Inport  Port=4
  SchliessZustand_LED_In : Inport  Port=5
  AlarmZustand_LED_In : Inport  Port=6
  CanData_Alarm_1_In : Inport  Port=7
  CanTrigger_Alarm_1_In : Inport  Port=8
  CanData_Schloss_1_In : Inport  Port=9
  CanTrigger_Schloss_1_In : Inport  Port=10
  Bus Creator : BusCreator  Inputs=6
  CanBus_Output : Subsystem
  CanTransmit_Alarm_1 : Subsystem
  CanTransmit_Schloss_1 : Subsystem
  SchlossAlarmLEDs : Subsystem
  CanBus_SA_Out : Outport
  tag scope: alarmOutputBus=global
  wires:
  CanData_Alarm_1_In/1 -> CanTransmit_Alarm_1/1(CanData_Alarm_1_In)  "CanData_Alarm_1"
  CanTransmit_Alarm_1/1(CanMsg_Alarm_1_Out) -> CanBus_Output/1(CanMsg_Alarm_1_In)  "CanMsg_Alarm_1"
  CanTrigger_Schloss_1_In/1 -> CanTransmit_Schloss_1/2(CanTrigger_Schloss_1_In)  "CanTrigger_Schloss_1"
  AlarmZustand_LED_In/1 -> Bus Creator/6, SchlossAlarmLEDs/2(Alarm_LED)  "AlarmZustand"
  CanBus_Output/1(CanBus_SA_Out) -> CanBus_SA_Out/1
  CanData_Schloss_1_In/1 -> CanTransmit_Schloss_1/1(CanData_Schloss_1_In)  "CanData_Schloss_1"
  SchliessZustand_LED_In/1 -> Bus Creator/5, SchlossAlarmLEDs/1(Schloss_LED)  "SchliessZustand"
  CanTransmit_Schloss_1/1(CanMsg_Schloss_1_Out) -> CanBus_Output/2(CanMsg_Schloss_1_In)  "CanMsg_Schloss_1"
  CanTrigger_Alarm_1_In/1 -> CanTransmit_Alarm_1/2(CanTrigger_Alarm_1_In)  "CanTrigger_Alarm_1"
  Bus Creator/1 -> [alarmOutputBus]
  GenericLedOben_LED_In/1 -> Bus Creator/4
  GenericLedRechts_LED_In/1 -> Bus Creator/3
  GenericLedLinks_LED_In/1 -> Bus Creator/2
  GenericLedUnten_LED_In/1 -> Bus Creator/1

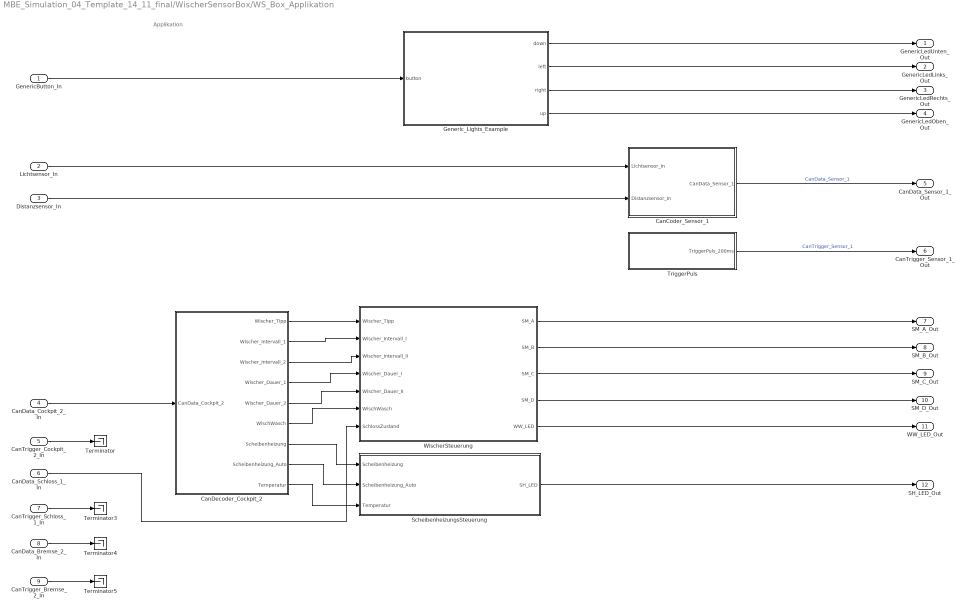
== system MBE_Simulation_04_Template_14_11_final/WischerSensorBox/WS_Box_Applikation ==
  note: Applikation
  GenericButton_In : Inport
  Lichtsensor_In : Inport  Port=2
  Distanzsensor_In : Inport  Port=3
  CanData_Cockpit_2_In : Inport  Port=4
  CanTrigger_Cockpit_2_In : Inport  Port=5
  CanData_Schloss_1_In : Inport  Port=6
  CanTrigger_Schloss_1_In : Inport  Port=7
  CanData_Bremse_2_In : Inport  Port=8
  CanTrigger_Bremse_2_In : Inport  Port=9
  CanCoder_Sensor_1 : Subsystem
  CanDecoder_Cockpit_2 : Subsystem
  Generic_Lights_Example : Stateflow chart  TreatAsAtomicUnit=on
  ScheibenheizungsSteuerung : Stateflow chart  TreatAsAtomicUnit=on
  Terminator{,3..5} (4 alike) : Terminator
  TriggerPuls : Subsystem
  WischerSteuerung : Stateflow chart  TreatAsAtomicUnit=on
  GenericLedUnten_Out : Outport
  GenericLedLinks_Out : Outport  Port=2
  GenericLedRechts_Out : Outport  Port=3
  GenericLedOben_Out : Outport  Port=4
  CanData_Sensor_1_Out : Outport  Port=5
  CanTrigger_Sensor_1_Out : Outport  Port=6
  SM_A_Out : Outport  Port=7
  SM_B_Out : Outport  Port=8
  SM_C_Out : Outport  Port=9
  SM_D_Out : Outport  Port=10
  WW_LED_Out : Outport  Port=11
  SH_LED_Out : Outport  Port=12
  wires:
  ScheibenheizungsSteuerung/1(SH_LED) -> SH_LED_Out/1
  WischerSteuerung/3(SM_C) -> SM_C_Out/1
  WischerSteuerung/5(WW_LED) -> WW_LED_Out/1
  CanCoder_Sensor_1/1(CanData_Sensor_1) -> CanData_Sensor_1_Out/1  "CanData_Sensor_1"
  WischerSteuerung/1(SM_A) -> SM_A_Out/1
  WischerSteuerung/4(SM_D) -> SM_D_Out/1
  WischerSteuerung/2(SM_B) -> SM_B_Out/1
  Distanzsensor_In/1 -> CanCoder_Sensor_1/2(Distanzsensor_In)
  Lichtsensor_In/1 -> CanCoder_Sensor_1/1(Lichtsensor_In)
  CanTrigger_Cockpit_2_In/1 -> Terminator/1
  CanData_Cockpit_2_In/1 -> CanDecoder_Cockpit_2/1(CanData_Cockpit_2)
  CanDecoder_Cockpit_2/3(Wischer_Intervall_2) -> WischerSteuerung/3(Wischer_Intervall_II)
  CanDecoder_Cockpit_2/9(Temperatur) -> ScheibenheizungsSteuerung/3(Temperatur)
  CanDecoder_Cockpit_2/8(Scheibenheizung_Auto) -> ScheibenheizungsSteuerung/2(Scheibenheizung_Auto)
  CanDecoder_Cockpit_2/7(Scheibenheizung) -> ScheibenheizungsSteuerung/1(Scheibenheizung)
  CanDecoder_Cockpit_2/2(Wischer_Intervall_1) -> WischerSteuerung/2(Wischer_Intervall_I)
  CanDecoder_Cockpit_2/1(Wischer_Tipp) -> WischerSteuerung/1(Wischer_Tipp)
  CanDecoder_Cockpit_2/4(Wischer_Dauer_1) -> WischerSteuerung/4(Wischer_Dauer_I)
  CanDecoder_Cockpit_2/5(Wischer_Dauer_2) -> WischerSteuerung/5(Wischer_Dauer_II)
  CanDecoder_Cockpit_2/6(WischWasch) -> WischerSteuerung/6(WischWasch)
  CanTrigger_Bremse_2_In/1 -> Terminator5/1
  CanData_Bremse_2_In/1 -> Terminator4/1
  CanTrigger_Schloss_1_In/1 -> Terminator3/1
  Generic_Lights_Example/1(down) -> GenericLedUnten_Out/1
  Generic_Lights_Example/2(left) -> GenericLedLinks_Out/1
  Generic_Lights_Example/3(right) -> GenericLedRechts_Out/1
  Generic_Lights_Example/4(up) -> GenericLedOben_Out/1
  GenericButton_In/1 -> Generic_Lights_Example/1(button)
  TriggerPuls/1(TriggerPuls_200ms) -> CanTrigger_Sensor_1_Out/1  "CanTrigger_Sensor_1"
  CanData_Schloss_1_In/1 -> WischerSteuerung/7(SchlossZustand)

== system MBE_Simulation_04_Template_14_11_final/WischerSensorBox/WS_Box_Simulation_Input ==
  CanBus_WS_In : Inport
  CanBus_Input : Subsystem
  CanReceive_Bremse_2 : Subsystem
  CanReceive_Cockpit_2 : Subsystem
  CanReceive_Schloss_1 : Subsystem
  PanelInput_WischerSensorBox : Subsystem
  GenericButton_Out : Outport
  Lichtsensor_Out : Outport  Port=2
  Distanzsensor_Out : Outport  Port=3
  CanData_Cockpit_2_Out : Outport  Port=4
  CanTrigger_Cockpit_2_Out : Outport  Port=5
  CanData_Schloss_1_Out : Outport  Port=6
  CanTrigger_Schloss_1_Out : Outport  Port=7
  CanData_Bremse_2_Out : Outport  Port=8
  CanTrigger_Bremse_2_Out : Outport  Port=9
  wires:
  CanReceive_Bremse_2/1(CanData_Bremse_2_Out) -> CanData_Bremse_2_Out/1
  CanReceive_Bremse_2/2(CanTrigger_Bremse_2_Out) -> CanTrigger_Bremse_2_Out/1
  CanReceive_Schloss_1/2(CanTrigger_Schloss_1_Out) -> CanTrigger_Schloss_1_Out/1
  CanReceive_Schloss_1/1(CanData_Schloss_1_Out) -> CanData_Schloss_1_Out/1
  CanBus_Input/1(CanMsg_Cockpit_2_Out) -> CanReceive_Cockpit_2/1(CanMsg_Cockpit_2_In)
  CanReceive_Cockpit_2/2(CanTrigger_Cockpit_2_Out) -> CanTrigger_Cockpit_2_Out/1
  CanReceive_Cockpit_2/1(CanData_Cockpit_2_out) -> CanData_Cockpit_2_Out/1
  PanelInput_WischerSensorBox/3(DistanzSlider_Out) -> Distanzsensor_Out/1
  PanelInput_WischerSensorBox/2(LichtSwitch_Out) -> Lichtsensor_Out/1
  CanBus_WS_In/1 -> CanBus_Input/1(CanBus_WS_In)
  CanBus_Input/2(CanMsg_Schloss_1_Out) -> CanReceive_Schloss_1/1(CanMsg_Schloss_1_In)
  CanBus_Input/3(CanMsg_Bremse_2_Out) -> CanReceive_Bremse_2/1(CanMsg_Bremse_2_In)
  PanelInput_WischerSensorBox/1(GenericButton_Out) -> GenericButton_Out/1

== system MBE_Simulation_04_Template_14_11_final/WischerSensorBox/WS_Box_Simulation_Output ==
  GenericLedUnten_LED_In : Inport
  GenericLedLinks_LED_In : Inport  Port=2
  GenericLedRechts_LED_In : Inport  Port=3
  GenericLedOben_LED_In : Inport  Port=4
  CanData_Sensor_1_In : Inport  Port=5
  CanTrigger_Sensor_1_In : Inport  Port=6
  SM_A_In : Inport  Port=7
  SM_B_In : Inport  Port=8
  SM_C_In : Inport  Port=9
  SM_D_In : Inport  Port=10
  WW_LED_In : Inport  Port=11
  SH_LED_In : Inport  Port=12
  Bus Creator : BusCreator  Inputs=10
  CanBus_Output : Subsystem
  CanTransmit_Sensor_1 : Subsystem
  Schrittmotor : Subsystem
  WischerSensorLEDs : Subsystem
  CanBus_WS_Out : Outport
  tag scope: windshieldOutputBus=global
  wires:
  SM_D_In/1 -> Bus Creator/10, Schrittmotor/4(SM_D)
  CanTrigger_Sensor_1_In/1 -> CanTransmit_Sensor_1/2(CanTrigger_Sensor_1_In)  "CanTrigger_Sensor_1"
  CanData_Sensor_1_In/1 -> CanTransmit_Sensor_1/1(CanData_Sensor_1_In)  "CanData_Sensor_1"
  CanBus_Output/1(CanBus_WS_Out) -> CanBus_WS_Out/1
  SM_B_In/1 -> Bus Creator/8, Schrittmotor/2(SM_B)
  WW_LED_In/1 -> Bus Creator/6, WischerSensorLEDs/1(WW_LED)
  SM_C_In/1 -> Bus Creator/9, Schrittmotor/3(SM_C)
  SM_A_In/1 -> Bus Creator/7, Schrittmotor/1(SM_A)
  SH_LED_In/1 -> Bus Creator/5, WischerSensorLEDs/2(SH_LED)
  CanTransmit_Sensor_1/1(OutCanMsg_Sensor_1_Out) -> CanBus_Output/1(CanMsg_Sensor_1_In)
  Bus Creator/1 -> [windshieldOutputBus]
  GenericLedUnten_LED_In/1 -> Bus Creator/1
  GenericLedLinks_LED_In/1 -> Bus Creator/2
  GenericLedRechts_LED_In/1 -> Bus Creator/3
  GenericLedOben_LED_In/1 -> Bus Creator/4

== system MBE_Simulation_04_Template_14_11_final/Cockpit/CanCoder_Bremse_1/TriggerPuls ==
  Gain : Gain  Gain=2^0  OutDataTypeStr=uint8
  Pulse Generator : DiscretePulseGenerator  PulseType=Time based  Period=0.1  PulseWidth=50
  Scope : Scope
  TriggerPuls_100ms : Outport
  wires:
  Pulse Generator/1 -> Gain/1
  Gain/1 -> TriggerPuls_100ms/1, Scope/1

== system MBE_Simulation_04_Template_14_11_final/Cockpit/CanCoder_Cockpit_1/TriggerPuls ==
  Gain : Gain  Gain=2^0  OutDataTypeStr=uint8
  Pulse Generator : DiscretePulseGenerator  PulseType=Time based  Period=0.2  PulseWidth=50
  Scope : Scope
  TriggerPuls_200ms : Outport
  wires:
  Pulse Generator/1 -> Gain/1
  Gain/1 -> TriggerPuls_200ms/1, Scope/1

== system MBE_Simulation_04_Template_14_11_final/Cockpit/CanCoder_Cockpit_2/TriggerPuls ==
  Gain : Gain  Gain=2^0  OutDataTypeStr=uint8
  Pulse Generator : DiscretePulseGenerator  PulseType=Time based  Period=0.2  PulseWidth=50
  Scope : Scope
  TriggerPuls_200ms : Outport
  wires:
  Pulse Generator/1 -> Gain/1
  Gain/1 -> TriggerPuls_200ms/1, Scope/1

== system MBE_Simulation_04_Template_14_11_final/LeuchtenBlinkerBox/LB_Box_Applikation/CanDecoder_Alarm_1 ==
  CanData_Alarm_1 : Inport
  Compare To Constant1 : simulink/Logic and Bit Operations/Compare To Constant  relop=~=  const=0  OutDataTypeStr=boolean
  Extract Bits1 : simulink/Logic and Bit Operations/Extract Bits  bitsToExtract=Range of bits  numBits=8  bitIdxRange=[0 0]  outScalingMode=Treat bit field as an integer
      settings: SourceProductName=Simulink
  AlarmZustand : Outport
  wires:
  Compare To Constant1/1 -> AlarmZustand/1
  CanData_Alarm_1/1 -> Extract Bits1/1
  Extract Bits1/1 -> Compare To Constant1/1

== system MBE_Simulation_04_Template_14_11_final/LeuchtenBlinkerBox/LB_Box_Applikation/CanDecoder_Bremse_1 ==
  CanData_Bremse_1 : Inport
  Compare To Constant1 : simulink/Logic and Bit Operations/Compare To Constant  relop=~=  const=0  OutDataTypeStr=boolean
  Compare To Constant2 : simulink/Logic and Bit Operations/Compare To Constant  relop=~=  const=0  OutDataTypeStr=boolean
  Compare To Constant3 : simulink/Logic and Bit Operations/Compare To Constant  relop=~=  const=0  OutDataTypeStr=boolean
  Extract Bits1 : simulink/Logic and Bit Operations/Extract Bits  bitsToExtract=Range of bits  numBits=8  bitIdxRange=[0 0]  outScalingMode=Treat bit field as an integer
      settings: SourceProductName=Simulink
  Extract Bits2 : simulink/Logic and Bit Operations/Extract Bits  bitsToExtract=Range of bits  numBits=8  bitIdxRange=[1 1]  outScalingMode=Treat bit field as an integer
      settings: SourceProductName=Simulink
  Extract Bits3 : simulink/Logic and Bit Operations/Extract Bits  bitsToExtract=Range of bits  numBits=8  bitIdxRange=[2 2]  outScalingMode=Treat bit field as an integer
      settings: SourceProductName=Simulink
  Bremse : Outport
  WarnBremsung : Outport  Port=2
  NotBremsung : Outport  Port=3
  wires:
  Compare To Constant1/1 -> Bremse/1
  Extract Bits1/1 -> Compare To Constant1/1
  CanData_Bremse_1/1 -> Extract Bits1/1, Extract Bits3/1, Extract Bits2/1
  Compare To Constant2/1 -> WarnBremsung/1
  Extract Bits2/1 -> Compare To Constant2/1
  Compare To Constant3/1 -> NotBremsung/1
  Extract Bits3/1 -> Compare To Constant3/1

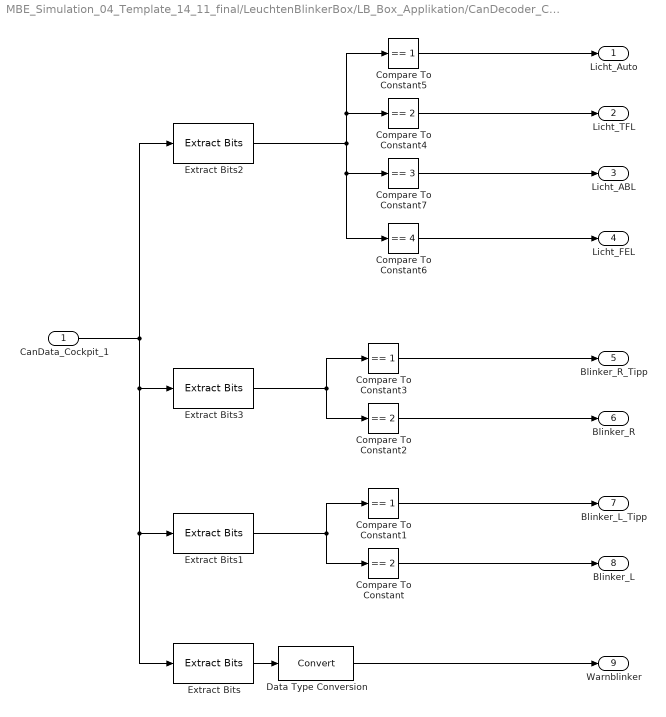
== system MBE_Simulation_04_Template_14_11_final/LeuchtenBlinkerBox/LB_Box_Applikation/CanDecoder_Cockpit_1 ==
  CanData_Cockpit_1 : Inport
  Compare To Constant : simulink/Logic and Bit Operations/Compare To Constant  relop===  const=2  OutDataTypeStr=boolean
  Compare To Constant1 : simulink/Logic and Bit Operations/Compare To Constant  relop===  const=1  OutDataTypeStr=boolean
  Compare To Constant2 : simulink/Logic and Bit Operations/Compare To Constant  relop===  const=2  OutDataTypeStr=boolean
  Compare To Constant3 : simulink/Logic and Bit Operations/Compare To Constant  relop===  const=1  OutDataTypeStr=boolean
  Compare To Constant4 : simulink/Logic and Bit Operations/Compare To Constant  relop===  const=2  OutDataTypeStr=boolean
  Compare To Constant5 : simulink/Logic and Bit Operations/Compare To Constant  relop===  const=1  OutDataTypeStr=boolean
  Compare To Constant6 : simulink/Logic and Bit Operations/Compare To Constant  relop===  const=4  OutDataTypeStr=boolean
  Compare To Constant7 : simulink/Logic and Bit Operations/Compare To Constant  relop===  const=3  OutDataTypeStr=boolean
  Data Type Conversion : DataTypeConversion
  Extract Bits : simulink/Logic and Bit Operations/Extract Bits  bitsToExtract=Range of bits  numBits=8  bitIdxRange=[7 7]  outScalingMode=Treat bit field as an integer
      settings: SourceProductName=Simulink
  Extract Bits1 : simulink/Logic and Bit Operations/Extract Bits  bitsToExtract=Range of bits  numBits=8  bitIdxRange=[5 6]  outScalingMode=Treat bit field as an integer
      settings: SourceProductName=Simulink
  Extract Bits2 : simulink/Logic and Bit Operations/Extract Bits  bitsToExtract=Range of bits  numBits=8  bitIdxRange=[0 2]  outScalingMode=Treat bit field as an integer
      settings: SourceProductName=Simulink
  Extract Bits3 : simulink/Logic and Bit Operations/Extract Bits  bitsToExtract=Range of bits  numBits=8  bitIdxRange=[3 4]  outScalingMode=Treat bit field as an integer
      settings: SourceProductName=Simulink
  Licht_Auto : Outport
  Licht_TFL : Outport  Port=2
  Licht_ABL : Outport  Port=3
  Licht_FEL : Outport  Port=4
  Blinker_R_Tipp : Outport  Port=5
  Blinker_R : Outport  Port=6
  Blinker_L_Tipp : Outport  Port=7
  Blinker_L : Outport  Port=8
  Warnblinker : Outport  Port=9
  wires:
  Extract Bits/1 -> Data Type Conversion/1
  Data Type Conversion/1 -> Warnblinker/1
  CanData_Cockpit_1/1 -> Extract Bits2/1, Extract Bits3/1, Extract Bits/1, Extract Bits1/1
  Compare To Constant/1 -> Blinker_L/1
  Compare To Constant1/1 -> Blinker_L_Tipp/1
  Extract Bits1/1 -> Compare To Constant/1, Compare To Constant1/1
  Extract Bits3/1 -> Compare To Constant2/1, Compare To Constant3/1
  Compare To Constant3/1 -> Blinker_R_Tipp/1
  Compare To Constant2/1 -> Blinker_R/1
  Extract Bits2/1 -> Compare To Constant6/1, Compare To Constant7/1, Compare To Constant5/1, Compare To Constant4/1
  Compare To Constant5/1 -> Licht_Auto/1
  Compare To Constant4/1 -> Licht_TFL/1
  Compare To Constant7/1 -> Licht_ABL/1
  Compare To Constant6/1 -> Licht_FEL/1

== system MBE_Simulation_04_Template_14_11_final/LeuchtenBlinkerBox/LB_Box_Applikation/CanDecoder_Schloss_1 ==
  CanData_Schloss_1 : Inport
  Compare To Constant1 : simulink/Logic and Bit Operations/Compare To Constant  relop=~=  const=0  OutDataTypeStr=boolean
  Extract Bits1 : simulink/Logic and Bit Operations/Extract Bits  bitsToExtract=Range of bits  numBits=8  bitIdxRange=[0 0]  outScalingMode=Treat bit field as an integer
      settings: SourceProductName=Simulink
  SchliessZustand : Outport
  wires:
  CanData_Schloss_1/1 -> Extract Bits1/1
  Compare To Constant1/1 -> SchliessZustand/1
  Extract Bits1/1 -> Compare To Constant1/1

== system MBE_Simulation_04_Template_14_11_final/LeuchtenBlinkerBox/LB_Box_Applikation/CanDecoder_Sensor_1 ==
  CanMsg_Sensor_1 : Inport
  Compare To Constant1 : simulink/Logic and Bit Operations/Compare To Constant  relop===  const=0  OutDataTypeStr=boolean
  Data Type Conversion : DataTypeConversion
  Data Type Conversion1 : DataTypeConversion  OutDataTypeStr=uint16
  Data Type Conversion2 : DataTypeConversion  OutDataTypeStr=uint16
  Extract Bits : simulink/Logic and Bit Operations/Extract Bits  bitsToExtract=Range of bits  numBits=8  bitIdxRange=[1 9]  outScalingMode=Treat bit field as an integer
      settings: SourceProductName=Simulink
  Extract Bits1 : simulink/Logic and Bit Operations/Extract Bits  bitsToExtract=Range of bits  numBits=1  bitIdxRange=[0 0]  outScalingMode=Treat bit field as an integer
      settings: SourceProductName=Simulink
  Helligkeit : Outport
  Distanz : Outport  Port=2
  wires:
  Extract Bits1/1 -> Data Type Conversion/1
  Data Type Conversion/1 -> Compare To Constant1/1
  Compare To Constant1/1 -> Helligkeit/1
  Extract Bits/1 -> Data Type Conversion1/1
  Data Type Conversion1/1 -> Distanz/1
  CanMsg_Sensor_1/1 -> Data Type Conversion2/1
  Data Type Conversion2/1 -> Extract Bits/1, Extract Bits1/1

== system MBE_Simulation_04_Template_14_11_final/LeuchtenBlinkerBox/LB_Box_Simulation_Input/CanBus_Input ==
  CanBus_LB_In : Inport
  Bus Selector3 : BusSelector  OutputSignals=CanBus_Cockpit.CanMsg_Cockpit_1,CanBus_SA.CanMsg_Schloss_1,CanBus_SA.CanMsg_Alarm_1,CanBus_WS.CanMsg_Sensor_1,CanBus_Cockpit.CanMsg_Bremse_1
  CanMsg_Cockpit_1_Out : Outport
  CanMsg_Schloss_1_Out : Outport  Port=2
  CanMsg_Alarm_1_Out : Outport  Port=3
  CanMsg_Sensor_1_Out : Outport  Port=4
  CanMsg_Bremse_1_Out : Outport  Port=5
  wires:
  CanBus_LB_In/1 -> Bus Selector3/1
  Bus Selector3/5 -> CanMsg_Bremse_1_Out/1  "<CanMsg_Bremse_1>"
  Bus Selector3/4 -> CanMsg_Sensor_1_Out/1  "<CanMsg_Sensor_1>"
  Bus Selector3/1 -> CanMsg_Cockpit_1_Out/1  "<CanMsg_Cockpit_1>"
  Bus Selector3/2 -> CanMsg_Schloss_1_Out/1  "<CanMsg_Schloss_1>"
  Bus Selector3/3 -> CanMsg_Alarm_1_Out/1  "<CanMsg_Alarm_1>"

== system MBE_Simulation_04_Template_14_11_final/LeuchtenBlinkerBox/LB_Box_Simulation_Input/CanReceive_Alarm_1 ==
  CanMsg_Alarm_1_In : Inport
  Bus Selector1 : BusSelector  OutputSignals=CanData_Alarm_1,CanTrigger_Alarm_1
  Detect Change4 : simulink/Logic and Bit Operations/Detect Change  vinit=0  OutDataTypeStr=boolean
  Terminator5 : Terminator
  CanData_Alarm_1_Out : Outport
  CanTrigger_Alarm_1_Out : Outport  Port=2
  wires:
  Bus Selector1/1 -> Detect Change4/1, CanData_Alarm_1_Out/1  "<CanData_Alarm_1>"
  Bus Selector1/2 -> Terminator5/1  "<CanTrigger_Alarm_1>"
  CanMsg_Alarm_1_In/1 -> Bus Selector1/1
  Detect Change4/1 -> CanTrigger_Alarm_1_Out/1

== system MBE_Simulation_04_Template_14_11_final/LeuchtenBlinkerBox/LB_Box_Simulation_Input/CanReceive_Bremse_1 ==
  CanMsg_Bremse_1_In : Inport
  Bus Selector5 : BusSelector  OutputSignals=CanData_Bremse_1,CanTrigger_Bremse_1
  Detect Change4 : simulink/Logic and Bit Operations/Detect Change  vinit=0  OutDataTypeStr=boolean
  Terminator8 : Terminator
  CanData_Bremse_1_Out : Outport
  CanTrigger_Bremse_1_Out : Outport  Port=2
  wires:
  Bus Selector5/1 -> Detect Change4/1, CanData_Bremse_1_Out/1  "<CanData_Bremse_1>"
  Bus Selector5/2 -> Terminator8/1  "<CanTrigger_Bremse_1>"
  Detect Change4/1 -> CanTrigger_Bremse_1_Out/1
  CanMsg_Bremse_1_In/1 -> Bus Selector5/1
